simulink model "Two_Zone_MVDC_PSolver"  (R2025b)
settings: Solver=FixedStepDiscrete  StartTime=0.0  StopTime=30  FixedStep=TsELEC  RelTol=1e-3  EnableMultiTasking=on
InitFcn:
  | TsELEC = 25e-6;
  | Ts = 25e-6;
undefined symbols (not defined in the file or in its folder): DiscIntNeverNeededParam, ee_sli_rtmsupport, GABDA, GABDB, GBBDA, GBBDB, gcbh, GPPMA, GPPMB, GPPMC, SADA, SADB, SADC, SADD, SBDA, SBDB, SBDC, SCDA, SCDB, SCDC, SCDD, SDDA, SDDB, SDDC, SDDD, SDDE, TsCont
libraries: fl_lib x97, nesl_utility x73, ee_lib x48, simulink x3, slpidlib x3, eeSmAC1C x2, eePowerMeasurement x2, mcbeeMathTransformLib x2, eeTransforms x1
(part 3 of 4)

== system Two_Zone_MVDC_PSolver/PMM/Control ==
  Selector : Selector  InputPortWidth=2  IndexOptions=Index vector (dialog)  Indices=2  OutputSizes=1
  Selector1 : Selector  InputPortWidth=2  IndexOptions=Index vector (dialog)  Indices=1  OutputSizes=1
  Speed Control : Subsystem
  Torque Control : Subsystem
  Unit Delay1 : UnitDelay  SampleTime=Ts  HasFrameUpgradeWarning=on
  duty_cycle : Outport
  wires:
  Unit Delay1/1 -> duty_cycle/1
  [Nref1] -> Speed Control/1(Speed_Ref_PU)
  [pos_speed_1] -> Selector/1, Selector1/1
  Selector/1 -> Speed Control/2(Speed_Meas_PU)
  [Iab_meas1] -> Torque Control/2(Iab_Sim)
  Torque Control/1(Vabc_out_PU) -> Unit Delay1/1
  Selector1/1 -> Torque Control/3(Pos_Sim)
  Speed Control/1(IdqRef_PU) -> Torque Control/1(Idq_ref_PU)

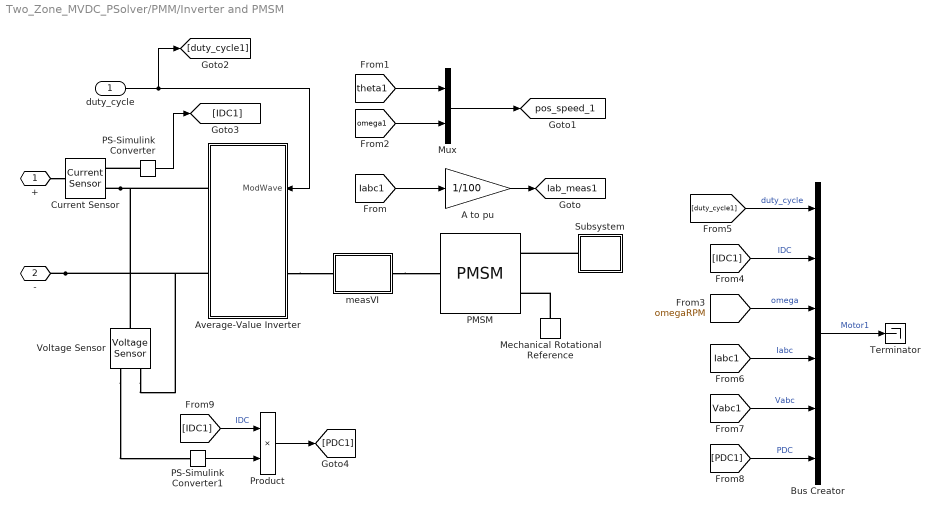
== system Two_Zone_MVDC_PSolver/PMM/Inverter and PMSM ==
  duty_cycle : Inport
  A to pu : Gain  Gain=1/100
  Average-Value Inverter : Subsystem
  Bus Creator : BusCreator  Inputs=6
  Current Sensor : fl_lib/Electrical/Electrical Sensors/Current Sensor
  Mechanical Rotational Reference : fl_lib/Mechanical/Rotational Elements/Mechanical Rotational Reference
  Mux : Mux  Inputs=2
  PMSM : ee_lib/Electromechanical/Permanent Magnet/PMSM  port_option=ee.enum.threePhasePort.composite  winding_type=ee.enum.statorconnection.wye  machine_param=ee.enum.pmsm.parameterization.constant  nPolePairs=1  pmflux_param=ee.enum.pmflux.fluxlinkage  pm_flux_linkage=3.15*4 Wb  torque_constant=0.18 N*m/A  back_emf_constant=0.18 V/(rad/s)  stator_param=ee.enum.statorparam.LdLqL0  Ld=0.0005 H  Lq=0.0009 H  idVec=[-200, 0, 200] A  iqVec=[-200, 0, 200] A  LdMatrix=0.0002 * ones(3, 3) H  LqMatrix=0.0002 * ones(3, 3) H  PmMatrix=0.1 * ones(3, 3) Wb  ktMatrix=0.18 * ones(3, 3) N*m/A  keMatrix=0.18 * ones(3, 3) V/(rad/s)  L0=0 H  Ls=0.0002 H  Lm=-0.00002 H  Ms=0.00002 H  Rs=0.001 Ohm  zero_sequence=ee.enum.park.zerosequence.exclude  axes_param=ee.enum.rotorangle.daxis  loss_param=ee.enum.ironloss.none  losses_oc=[0, 0, 0] W  losses_sc=[0, 0, 0] W  f_losses=60 Hz  Isc_losses=95 A  J=1 kg*m^2  lam=1 N*m/(rad/s)  i_d_specify=off  i_d_priority=None  i_d=0 A  i_d_nominal_specify=off  i_d_nominal_value=1  i_d_nominal_unit=A  i_q_specify=off  i_q_priority=None  i_q=0 A  i_q_nominal_specify=off  i_q_nominal_value=1  i_q_nominal_unit=A  torque_specify=off  torque_priority=None  torque=0 N*m  torque_nominal_specify=off  torque_nominal_value=1  torque_nominal_unit=N*m  angular_velocity_specify=off  angular_velocity_priority=High  angular_velocity=0 rpm  angular_velocity_nominal_specify=off  angular_velocity_nominal_value=1  angular_velocity_nominal_unit=rpm  angular_position_specify=off  angular_position_priority=High  angular_position=0 deg  angular_position_nominal_specify=off  angular_position_nominal_value=1  angular_position_nominal_unit=deg  alpha=3.93e-3 1/K  alpha_flux=-0.001 1/K  Tmeas=298.15 K  stator_thermal_mass=100 J/K  rotor_thermal_mass=200 J/K  Rm_percent_rotor=90  Rd_percent_rotor=30  temperatureA_specify=off  temperatureA_priority=High  temperatureA=25 degC  temperatureA_nominal_specify=off  temperatureA_nominal_value=1  temperatureA_nominal_unit=degC  temperatureB_specify=off  temperatureB_priority=High  temperatureB=25 degC  temperatureB_nominal_specify=off  temperatureB_nominal_value=1  temperatureB_nominal_unit=degC  temperatureC_specify=off  temperatureC_priority=High  temperatureC=25 degC  temperatureC_nominal_specify=off  temperatureC_nominal_value=1  temperatureC_nominal_unit=degC  temperatureR_specify=off  temperatureR_priority=High  temperatureR=25 degC  temperatureR_nominal_specify=off  temperatureR_nominal_value=1  temperatureR_nominal_unit=degC
      settings: InternalSimscapePortConfiguration="{\"Bottom\":[],\"Left\":[{\"id\":\"N\",\"label\":\"~\",\"type\":\"foundation.electrical.three_phase\"}],\"Right\":[{\"id\":\"R\",\"label\":\"R\",\"type\":\"foundation.mechanical.rotational.rotational\"},{\"id\":\"C\",\"label\":\"C\",\"type\":\"foundation.mechanical.rotational.rotational\"}],\"Top\":[]}"
  PS-Simulink Converter : nesl_utility/PS-Simulink Converter  PhysicalDomain=network_engine_domain  SubClassName=ps_output  LeftPortType=input  RightPortType=output  PseudoPeriodic=off  Frequencies=[]  VectorFormat=1-D array  Unit=inherit  AffineConversion=off
  PS-Simulink Converter1 : nesl_utility/PS-Simulink Converter  PhysicalDomain=network_engine_domain  SubClassName=ps_output  LeftPortType=input  RightPortType=output  PseudoPeriodic=off  Frequencies=[]  VectorFormat=1-D array  Unit=inherit  AffineConversion=off
  Product : Product
  Subsystem : Subsystem
  Terminator : Terminator
  Voltage Sensor : fl_lib/Electrical/Electrical Sensors/Voltage Sensor
  measVI : Subsystem
  + : PMIOPort  Side=Left
  - : PMIOPort  Port=2  Side=Left
  tag scope: Iab_meas1=global, pos_speed_1=global
  wires:
  duty_cycle/1 -> Average-Value Inverter/1(ModWave), [duty_cycle1]
  [IDC1] -> Product/1  "IDC"
  [PDC1] -> Bus Creator/6  "PDC"
  Product/1 -> [PDC1]
  PS-Simulink Converter1/1 -> Product/2
  A to pu/1 -> [Iab_meas1]
  [Iabc1] -> A to pu/1
  [theta1] -> Mux/1
  [omega1] -> Mux/2
  Mux/1 -> [pos_speed_1]
  PS-Simulink Converter/1 -> [IDC1]
  [duty_cycle1] -> Bus Creator/1  "duty_cycle"
  [IDC1] -> Bus Creator/2  "IDC"
  [omegaRPM] -> Bus Creator/3  "omega"
  Bus Creator/1 -> Terminator/1  "Motor1"
  [Iabc1] -> Bus Creator/4  "Iabc"
  [Vabc1] -> Bus Creator/5  "Vabc"
  connections:
  Voltage Sensor/RConn1 -- PS-Simulink Converter1/LConn1
  Mechanical Rotational Reference/LConn1 -- PMSM/RConn2
  Subsystem/RConn1 -- PMSM/RConn1
  Average-Value Inverter/LConn1 -- measVI/LConn1
  measVI/RConn1 -- PMSM/LConn1
  Current Sensor/RConn2 -- Voltage Sensor/LConn1 -- Average-Value Inverter/RConn1
  PS-Simulink Converter/LConn1 -- Current Sensor/RConn1
  +/RConn1 -- Current Sensor/LConn1
  -/RConn1 -- Voltage Sensor/RConn2 -- Average-Value Inverter/RConn2

== system Two_Zone_MVDC_PSolver/PMM/Speed Reference ==
  LPF : Subsystem
  Power Reference : simulink/Sources/Repeating Sequence Interpolated  OutValues=[0 0 0.5 0.5 -0.5 -0.5]  TimeValues=[0 5 10 15 25 100]  LookUpMeth=Interpolation-Use End Values  tsamp=TsELEC  OutMin=[]  OutMax=[]  OutDataTypeStr=double  OutputDataTypeScalingMode=double  OutDataType=fixdt(0,8)  OutScaling=2^-10
  tag scope: Nref1=global
  wires:
  Power Reference/1 -> LPF/1(u)
  LPF/1(y) -> [Nref1]

== system Two_Zone_MVDC_PSolver/PGM1/Gas turbine/ AC1C ==
  Constant1 : Constant  Value=0  SampleTime=TsCont
  Constant2 : Constant  Value=0  SampleTime=TsCont
  PS-Simulink Converter : nesl_utility/PS-Simulink Converter  PhysicalDomain=network_engine_domain  SubClassName=ps_output  LeftPortType=input  RightPortType=output  PseudoPeriodic=off  Frequencies=[]  VectorFormat=1-D array  Unit=inherit  AffineConversion=off
  PS-Simulink Converter1 : nesl_utility/PS-Simulink Converter  PhysicalDomain=network_engine_domain  SubClassName=ps_output  LeftPortType=input  RightPortType=output  PseudoPeriodic=off  Frequencies=[]  VectorFormat=1-D array  Unit=inherit  AffineConversion=off
  Rate Transition : RateTransition  OutPortSampleTime=TsELEC
  Rate Transition1 : RateTransition  OutPortSampleTime=TsCont
  Rate Transition2 : RateTransition  OutPortSampleTime=TsCont
  Repeating Sequence Interpolated2 : simulink/Sources/Repeating Sequence Interpolated  OutValues=[1 1 1]  TimeValues=[0 5 1000]  LookUpMeth=Interpolation-Use End Values  tsamp=TsCont  OutMin=[]  OutMax=[]  OutDataTypeStr=double  OutputDataTypeScalingMode=double  OutDataType=fixdt(0,8)  OutScaling=2^-10
  SM AC1C : eeSmAC1C/SM AC1C  E_FD0=1  Ts=TsCont  R_C=0  X_C=0  T_R=0  K_A=80  T_A=0.2  T_B=0  T_C=0  K_F=0.03  T_F=1.49  V_Amax=14.5  V_Amin=-14.5  E_FEmax=6.03  E_FEmin=-5.43  oelInputLocation=Unused  uelInputLocation=Unused  sclInputLocation=Unused  K_E=1  T_E=0.8  K_C=0.2  K_D=0.38  E_1=4.18  S_E_E1=0.1  E_2=3.14  S_E_E2=0.03  V_FEmax=99  V_Emin=0
      settings: LibrarySourceBlock=ee_sl_lib/SM Control/SM AC1C
  Simulink-PS Converter : nesl_utility/Simulink-PS Converter  PhysicalDomain=network_engine_domain  SubClassName=ps_input  LeftPortType=input  RightPortType=output  PseudoPeriodic=off  Frequencies=[]  NoiseDistribution=none  NoiseParameters=[]  Unit=1  AffineConversion=off  FilteringAndDerivatives=provide  SimscapeFilterOrder=1  InputFilterTimeConstant=0.001  UdotUserProvided=0
  Synchronous Machine Field Circuit (pu) : ee_lib/Electromechanical/Synchronous/Synchronous Machine Field Circuit  unit_option=ee.enum.unit.pu  SRated=36e6 V*A  FRated=60 Hz  fieldCircuitParameterization_option=ee.enum.sm.fieldparameterization.current  baseEfd=92.95 V  baseIfd=200 A  parameterization_option=ee.enum.sm.parameterization.standard  Ladu=1.66  Rfd=0.0006  Xl=0.15  Xd=1.81  Xdd=0.3  Xddd=0.23  d_option=ee.enum.circuit.open  Td0d=8 s  Tdd=1.3260 s  Td0dd=0.03 s  Tddd=0.0230 s
      settings: LogSimulationData=on  InternalSimscapePortConfiguration="{\"Bottom\":[],\"Left\":[{\"id\":\"Efd_pu\",\"label\":\"Efd_pu\",\"type\":\"input\"},{\"id\":\"Ifd_pu\",\"label\":\"Ifd_pu\",\"type\":\"output\"}],\"Right\":[{\"id\":\"fd_p\",\"label\":\"fd+\",\"type\":\"foundation.electrical.electrical\"},{\"id\":\"fd_n\",\"label\":\"fd-\",\"type\":\"foundation.electrical.electrical\"}],\"Top\":[]}"
  Terminal Voltage Measurement : ee_lib/Electromechanical/Synchronous/Synchronous Machine Measurement  output_idx=14
      settings: LogSimulationData=on  InternalSimscapePortConfiguration="{\"Bottom\":[],\"Left\":[{\"id\":\"pu_input\",\"label\":\"pu\",\"type\":\"input\"}],\"Right\":[{\"id\":\"pu_output\",\"label\":\"o\",\"type\":\"output\"}],\"Top\":[]}"
  Unit Delay : UnitDelay  InitialCondition=1.37673  SampleTime=-1  HasFrameUpgradeWarning=on
  pu : PMIOPort  Side=Left
  fd+ : PMIOPort  Port=2  Side=Right
  fd- : PMIOPort  Port=3  Side=Right
  wires:
  PS-Simulink Converter1/1 -> Unit Delay/1
  PS-Simulink Converter/1 -> Rate Transition1/1  "Vt1"
  Unit Delay/1 -> Rate Transition2/1  "Ifd1"
  Rate Transition/1 -> Simulink-PS Converter/1
  Repeating Sequence Interpolated2/1 -> SM AC1C/1
  Constant1/1 -> SM AC1C/2
  Rate Transition2/1 -> SM AC1C/10
  Rate Transition1/1 -> SM AC1C/3
  Constant2/1 -> SM AC1C/8, SM AC1C/7, SM AC1C/6, SM AC1C/5, SM AC1C/4, SM AC1C/9
  SM AC1C/1 -> Rate Transition/1
  connections:
  fd-/RConn1 -- Synchronous Machine Field Circuit (pu)/RConn2
  Synchronous Machine Field Circuit (pu)/RConn1 -- fd+/RConn1
  PS-Simulink Converter1/LConn1 -- Synchronous Machine Field Circuit (pu)/LConn2
  Simulink-PS Converter/RConn1 -- Synchronous Machine Field Circuit (pu)/LConn1
  pu/RConn1 -- Terminal Voltage Measurement/LConn1
  PS-Simulink Converter/LConn1 -- Terminal Voltage Measurement/RConn1

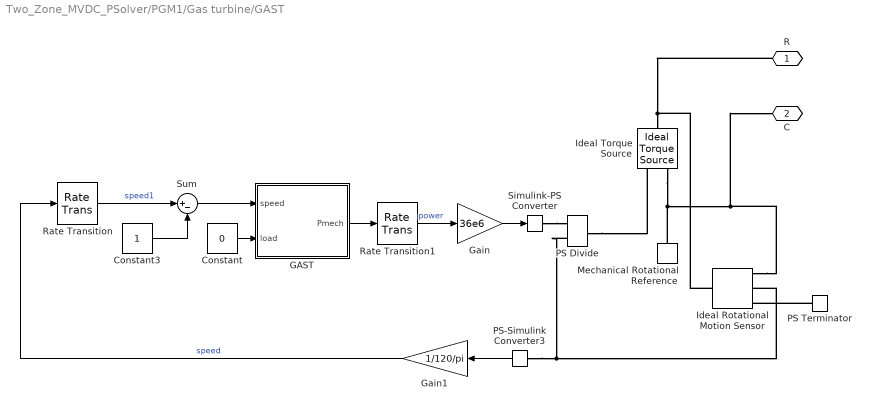
== system Two_Zone_MVDC_PSolver/PGM1/Gas turbine/GAST ==
  Constant : Constant  Value=0  SampleTime=TsCont
  Constant3 : Constant  SampleTime=TsCont
  GAST : Subsystem  mask{R=0.01, T1=0.005, T2=0.04, T3=0.1, AT=0.9, Kt=2, Vmax=1, Vmin=0, Dturb=0.03}
  Gain : Gain  Gain=36e6
  Gain1 : Gain  Gain=1/120/pi
  Ideal Rotational Motion Sensor : fl_lib/Mechanical/Mechanical Sensors/Ideal Rotational Motion Sensor  reference=foundation.enum.MeasurementReference.difference  acceleration_port=false  velocity_port=true  position_port=true  wrap_angle=simscape.enum.onoff.off  offset=0 rad
  Ideal Torque Source : fl_lib/Mechanical/Mechanical Sources/Ideal Torque Source
  Mechanical Rotational Reference : fl_lib/Mechanical/Rotational Elements/Mechanical Rotational Reference
  PS Divide : fl_lib/Physical Signals/Functions/PS Divide
  PS Terminator : fl_lib/Physical Signals/Sinks/PS Terminator
  PS-Simulink Converter3 : nesl_utility/PS-Simulink Converter  PhysicalDomain=network_engine_domain  SubClassName=ps_output  LeftPortType=input  RightPortType=output  PseudoPeriodic=off  Frequencies=[]  VectorFormat=1-D array  Unit=inherit  AffineConversion=off
  Rate Transition : RateTransition  Deterministic=off  OutPortSampleTime=TsCont
  Rate Transition1 : RateTransition  Deterministic=off  InitialCondition=2000/3/60*2*pi  OutPortSampleTime=Ts
  Simulink-PS Converter : nesl_utility/Simulink-PS Converter  PhysicalDomain=network_engine_domain  SubClassName=ps_input  LeftPortType=input  RightPortType=output  PseudoPeriodic=off  Frequencies=[]  NoiseDistribution=none  NoiseParameters=[]  Unit=W  AffineConversion=off  FilteringAndDerivatives=provide  SimscapeFilterOrder=1  InputFilterTimeConstant=0.001  UdotUserProvided=0
  Sum : Sum  Inputs=|+-
  R : PMIOPort  Side=Right
  C : PMIOPort  Port=2  Side=Right
  wires:
  Constant3/1 -> Sum/2
  Gain1/1 -> Rate Transition/1  "speed"
  GAST/1(Pmech) -> Rate Transition1/1
  Constant/1 -> GAST/2(load)
  Rate Transition1/1 -> Gain/1  "power"
  Rate Transition/1 -> Sum/1  "speed1"
  Sum/1 -> GAST/1(speed)
  Gain/1 -> Simulink-PS Converter/1
  PS-Simulink Converter3/1 -> Gain1/1
  connections:
  Ideal Rotational Motion Sensor/RConn2 -- PS-Simulink Converter3/LConn1 -- PS Divide/LConn2
  PS Terminator/LConn1 -- Ideal Rotational Motion Sensor/RConn3
  Ideal Torque Source/RConn2 -- Mechanical Rotational Reference/LConn1 -- C/RConn1 -- Ideal Rotational Motion Sensor/RConn1
  PS Divide/RConn1 -- Ideal Torque Source/RConn1
  Simulink-PS Converter/RConn1 -- PS Divide/LConn1
  R/RConn1 -- Ideal Rotational Motion Sensor/LConn1 -- Ideal Torque Source/LConn1

== system Two_Zone_MVDC_PSolver/PGM2/Gas turbine/ AC1C ==
  Constant1 : Constant  Value=0  SampleTime=TsCont
  Constant2 : Constant  Value=0  SampleTime=TsCont
  PS-Simulink Converter : nesl_utility/PS-Simulink Converter  PhysicalDomain=network_engine_domain  SubClassName=ps_output  LeftPortType=input  RightPortType=output  PseudoPeriodic=off  Frequencies=[]  VectorFormat=1-D array  Unit=inherit  AffineConversion=off
  PS-Simulink Converter1 : nesl_utility/PS-Simulink Converter  PhysicalDomain=network_engine_domain  SubClassName=ps_output  LeftPortType=input  RightPortType=output  PseudoPeriodic=off  Frequencies=[]  VectorFormat=1-D array  Unit=inherit  AffineConversion=off
  Rate Transition : RateTransition  OutPortSampleTime=TsELEC
  Rate Transition1 : RateTransition  OutPortSampleTime=TsCont
  Rate Transition2 : RateTransition  OutPortSampleTime=TsCont
  Repeating Sequence Interpolated2 : simulink/Sources/Repeating Sequence Interpolated  OutValues=[1 1 1]  TimeValues=[0 5 1000]  LookUpMeth=Interpolation-Use End Values  tsamp=TsCont  OutMin=[]  OutMax=[]  OutDataTypeStr=double  OutputDataTypeScalingMode=double  OutDataType=fixdt(0,8)  OutScaling=2^-10
  SM AC1C : eeSmAC1C/SM AC1C  E_FD0=1  Ts=TsCont  R_C=0  X_C=0  T_R=0  K_A=80  T_A=0.2  T_B=0  T_C=0  K_F=0.03  T_F=1.49  V_Amax=14.5  V_Amin=-14.5  E_FEmax=6.03  E_FEmin=-5.43  oelInputLocation=Unused  uelInputLocation=Unused  sclInputLocation=Unused  K_E=1  T_E=0.8  K_C=0.2  K_D=0.38  E_1=4.18  S_E_E1=0.1  E_2=3.14  S_E_E2=0.03  V_FEmax=99  V_Emin=0
      settings: LibrarySourceBlock=ee_sl_lib/SM Control/SM AC1C
  Simulink-PS Converter : nesl_utility/Simulink-PS Converter  PhysicalDomain=network_engine_domain  SubClassName=ps_input  LeftPortType=input  RightPortType=output  PseudoPeriodic=off  Frequencies=[]  NoiseDistribution=none  NoiseParameters=[]  Unit=1  AffineConversion=off  FilteringAndDerivatives=provide  SimscapeFilterOrder=1  InputFilterTimeConstant=0.001  UdotUserProvided=0
  Synchronous Machine Field Circuit (pu) : ee_lib/Electromechanical/Synchronous/Synchronous Machine Field Circuit  unit_option=ee.enum.unit.pu  SRated=36e6 V*A  FRated=60 Hz  fieldCircuitParameterization_option=ee.enum.sm.fieldparameterization.current  baseEfd=92.95 V  baseIfd=200 A  parameterization_option=ee.enum.sm.parameterization.standard  Ladu=1.66  Rfd=0.0006  Xl=0.15  Xd=1.81  Xdd=0.3  Xddd=0.23  d_option=ee.enum.circuit.open  Td0d=8 s  Tdd=1.3260 s  Td0dd=0.03 s  Tddd=0.0230 s
      settings: LogSimulationData=on  InternalSimscapePortConfiguration="{\"Bottom\":[],\"Left\":[{\"id\":\"Efd_pu\",\"label\":\"Efd_pu\",\"type\":\"input\"},{\"id\":\"Ifd_pu\",\"label\":\"Ifd_pu\",\"type\":\"output\"}],\"Right\":[{\"id\":\"fd_p\",\"label\":\"fd+\",\"type\":\"foundation.electrical.electrical\"},{\"id\":\"fd_n\",\"label\":\"fd-\",\"type\":\"foundation.electrical.electrical\"}],\"Top\":[]}"
  Terminal Voltage Measurement : ee_lib/Electromechanical/Synchronous/Synchronous Machine Measurement  output_idx=14
      settings: LogSimulationData=on  InternalSimscapePortConfiguration="{\"Bottom\":[],\"Left\":[{\"id\":\"pu_input\",\"label\":\"pu\",\"type\":\"input\"}],\"Right\":[{\"id\":\"pu_output\",\"label\":\"o\",\"type\":\"output\"}],\"Top\":[]}"
  Unit Delay : UnitDelay  InitialCondition=1.37673  SampleTime=-1  HasFrameUpgradeWarning=on
  pu : PMIOPort  Side=Left
  fd+ : PMIOPort  Port=2  Side=Right
  fd- : PMIOPort  Port=3  Side=Right
  wires:
  SM AC1C/1 -> Rate Transition/1
  PS-Simulink Converter1/1 -> Unit Delay/1
  Repeating Sequence Interpolated2/1 -> SM AC1C/1
  PS-Simulink Converter/1 -> Rate Transition1/1  "Vt1"
  Unit Delay/1 -> Rate Transition2/1  "Ifd1"
  Constant1/1 -> SM AC1C/2
  Rate Transition/1 -> Simulink-PS Converter/1
  Rate Transition1/1 -> SM AC1C/3
  Rate Transition2/1 -> SM AC1C/10
  Constant2/1 -> SM AC1C/8, SM AC1C/7, SM AC1C/6, SM AC1C/5, SM AC1C/4, SM AC1C/9
  connections:
  fd-/RConn1 -- Synchronous Machine Field Circuit (pu)/RConn2
  Synchronous Machine Field Circuit (pu)/RConn1 -- fd+/RConn1
  PS-Simulink Converter1/LConn1 -- Synchronous Machine Field Circuit (pu)/LConn2
  Simulink-PS Converter/RConn1 -- Synchronous Machine Field Circuit (pu)/LConn1
  pu/RConn1 -- Terminal Voltage Measurement/LConn1
  PS-Simulink Converter/LConn1 -- Terminal Voltage Measurement/RConn1

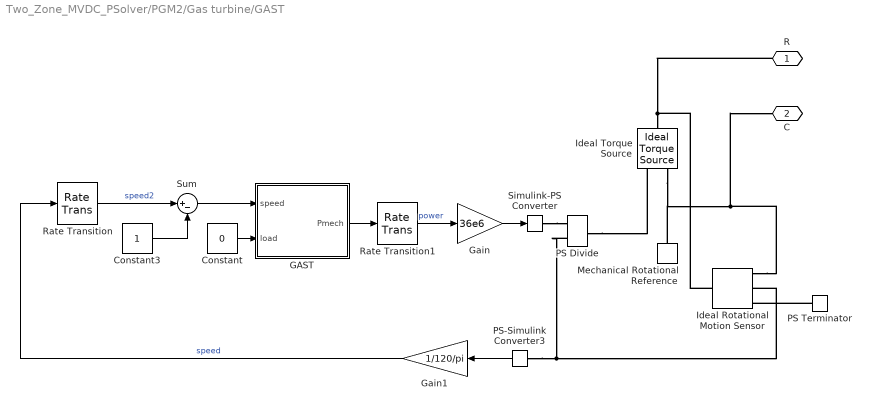
== system Two_Zone_MVDC_PSolver/PGM2/Gas turbine/GAST ==
  Constant : Constant  Value=0  SampleTime=TsCont
  Constant3 : Constant  SampleTime=TsCont
  GAST : Subsystem  mask{R=0.01, T1=0.005, T2=0.04, T3=0.1, AT=0.9, Kt=2, Vmax=1, Vmin=0, Dturb=0.03}
  Gain : Gain  Gain=36e6
  Gain1 : Gain  Gain=1/120/pi
  Ideal Rotational Motion Sensor : fl_lib/Mechanical/Mechanical Sensors/Ideal Rotational Motion Sensor  reference=foundation.enum.MeasurementReference.difference  acceleration_port=false  velocity_port=true  position_port=true  wrap_angle=simscape.enum.onoff.off  offset=0 rad
  Ideal Torque Source : fl_lib/Mechanical/Mechanical Sources/Ideal Torque Source
  Mechanical Rotational Reference : fl_lib/Mechanical/Rotational Elements/Mechanical Rotational Reference
  PS Divide : fl_lib/Physical Signals/Functions/PS Divide
  PS Terminator : fl_lib/Physical Signals/Sinks/PS Terminator
  PS-Simulink Converter3 : nesl_utility/PS-Simulink Converter  PhysicalDomain=network_engine_domain  SubClassName=ps_output  LeftPortType=input  RightPortType=output  PseudoPeriodic=off  Frequencies=[]  VectorFormat=1-D array  Unit=inherit  AffineConversion=off
  Rate Transition : RateTransition  Deterministic=off  OutPortSampleTime=TsCont
  Rate Transition1 : RateTransition  Deterministic=off  InitialCondition=2000/3/60*2*pi  OutPortSampleTime=Ts
  Simulink-PS Converter : nesl_utility/Simulink-PS Converter  PhysicalDomain=network_engine_domain  SubClassName=ps_input  LeftPortType=input  RightPortType=output  PseudoPeriodic=off  Frequencies=[]  NoiseDistribution=none  NoiseParameters=[]  Unit=W  AffineConversion=off  FilteringAndDerivatives=provide  SimscapeFilterOrder=1  InputFilterTimeConstant=0.001  UdotUserProvided=0
  Sum : Sum  Inputs=|+-
  R : PMIOPort  Side=Right
  C : PMIOPort  Port=2  Side=Right
  wires:
  Constant3/1 -> Sum/2
  Gain1/1 -> Rate Transition/1  "speed"
  GAST/1(Pmech) -> Rate Transition1/1
  Constant/1 -> GAST/2(load)
  Rate Transition1/1 -> Gain/1  "power"
  Rate Transition/1 -> Sum/1  "speed2"
  Sum/1 -> GAST/1(speed)
  Gain/1 -> Simulink-PS Converter/1
  PS-Simulink Converter3/1 -> Gain1/1
  connections:
  PS Divide/LConn2 -- Ideal Rotational Motion Sensor/RConn2 -- PS-Simulink Converter3/LConn1
  PS Terminator/LConn1 -- Ideal Rotational Motion Sensor/RConn3
  Ideal Rotational Motion Sensor/RConn1 -- Mechanical Rotational Reference/LConn1 -- Ideal Torque Source/RConn2 -- C/RConn1
  PS Divide/RConn1 -- Ideal Torque Source/RConn1
  Simulink-PS Converter/RConn1 -- PS Divide/LConn1
  R/RConn1 -- Ideal Torque Source/LConn1 -- Ideal Rotational Motion Sensor/LConn1

== system Two_Zone_MVDC_PSolver/PMM/Control/Speed Control ==
  Speed_Ref_PU : Inport
  Speed_Meas_PU : Inport  Port=2
  Id_ref : Constant  Value=0  OutDataTypeStr=Inherit: Inherit via back propagation  SampleTime=Ts
  Mux1 : Mux  Inputs=2
  PI_Controller_Speed : Subsystem
  IdqRef_PU : Outport  VectorParamsAs1DForOutWhenUnconnected=off
  wires:
  PI_Controller_Speed/1(Iq_ref) -> Mux1/2
  Id_ref/1 -> Mux1/1
  Speed_Ref_PU/1 -> PI_Controller_Speed/1(N_ref)
  Speed_Meas_PU/1 -> PI_Controller_Speed/2(N_fb)
  Mux1/1 -> IdqRef_PU/1

== system Two_Zone_MVDC_PSolver/PMM/Control/Torque Control ==
  Idq_ref_PU : Inport
  Iab_Sim : Inport  Port=2
  Pos_Sim : Inport  Port=3
  Control_System : Subsystem
  Gain : Gain
  Selector : Selector  InputPortWidth=3  IndexOptions=Index vector (dialog)  Indices=[1 2]  OutputSizes=1
  Vabc_out_PU : Outport  VectorParamsAs1DForOutWhenUnconnected=off
  wires:
  Selector/1 -> Control_System/1(Iab_meas_PU)
  Control_System/1(Vabc in PU) -> Vabc_out_PU/1
  Pos_Sim/1 -> Gain/1
  Iab_Sim/1 -> Selector/1
  Idq_ref_PU/1 -> Control_System/3(Idq_ref_PU)
  Gain/1 -> Control_System/2(Pos_PU)

== system Two_Zone_MVDC_PSolver/PMM/Inverter and PMSM/Average-Value Inverter ==
  ModWave : Inport
  Average-Value Voltage Source Converter (Three-Phase) : ee_lib/Semiconductors & Converters/Converters/Average-Value Voltage Source Converter (Three-Phase)  port_option=ee.enum.threePhasePort.composite  frequency_option=ee.enum.converters.frequency.variable  input_option=ee.enum.converters.inputOption.ModWave  FRated=60 Hz  losses_parameterization=ee.enum.converters.losses.fixed  Pfixed=1 W  ks=0.01  kc1=1.7 V  kc2=0.01 Ohm  Ploss_vect=[100, 800, 1870, 3250, 4900] W  Irms_vect=[10, 100, 200, 300, 400] A  Vdc_nom=300 V  thermal_mass=30000 J/K  temperature_specify=off  temperature_priority=High  temperature=298.15 K  temperature_nominal_specify=off  temperature_nominal_value=1  temperature_nominal_unit=K
      settings: InternalSimscapePortConfiguration="{\"Bottom\":[],\"Left\":[{\"id\":\"ModWave\",\"label\":\"ModWave\",\"type\":\"input\"},{\"id\":\"N\",\"label\":\"~\",\"type\":\"foundation.electrical.three_phase\"}],\"Right\":[{\"id\":\"p\",\"label\":\"+\",\"type\":\"foundation.electrical.electrical\"},{\"id\":\"n\",\"label\":\"-\",\"type\":\"foundation.electrical.electrical\"}],\"Top\":[]}"
  Simulink-PS Converter : nesl_utility/Simulink-PS Converter  PhysicalDomain=network_engine_domain  SubClassName=ps_input  LeftPortType=input  RightPortType=output  PseudoPeriodic=off  Frequencies=[]  NoiseDistribution=none  NoiseParameters=[]  Unit=1  AffineConversion=off  FilteringAndDerivatives=zero  SimscapeFilterOrder=1  InputFilterTimeConstant=0.001  UdotUserProvided=0
  + : PMIOPort  Side=Right
  ~ : PMIOPort  Port=2  Side=Left
  - : PMIOPort  Port=3  Side=Right
  wires:
  ModWave/1 -> Simulink-PS Converter/1
  connections:
  Simulink-PS Converter/RConn1 -- Average-Value Voltage Source Converter (Three-Phase)/LConn1
  Average-Value Voltage Source Converter (Three-Phase)/RConn2 -- -/RConn1
  Average-Value Voltage Source Converter (Three-Phase)/RConn1 -- +/RConn1
  Average-Value Voltage Source Converter (Three-Phase)/LConn2 -- ~/RConn1

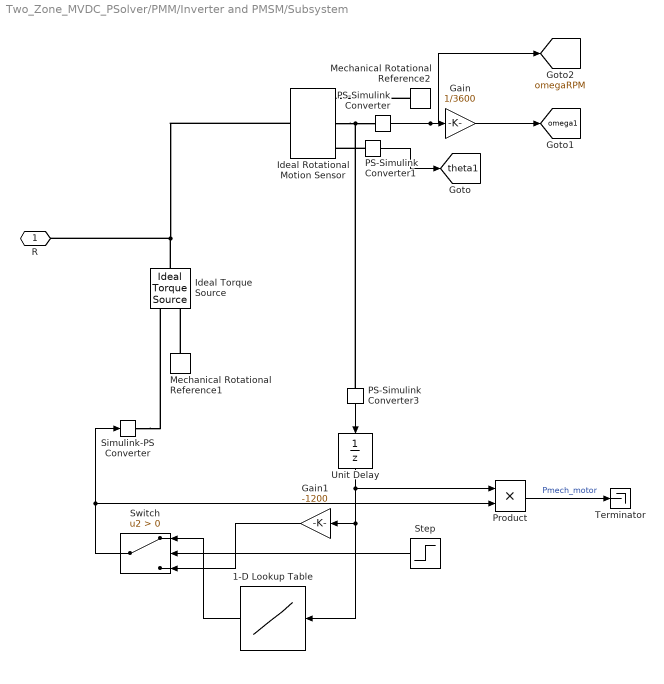
== system Two_Zone_MVDC_PSolver/PMM/Inverter and PMSM/Subsystem ==
  1-D Lookup Table : Lookup_n-D  NumberOfTableDimensions=1  BreakpointsForDimension1=[-120*pi 0 50*pi 120*pi]/2  Table=[120*pi*1200 50*pi*1200 0 -120*pi*1200]/2  InternalRulePriority=Speed  RndMeth=Simplest
  Gain : Gain  Gain=1/3600
  Gain1 : Gain  Gain=-1200
  Ideal Rotational Motion Sensor : fl_lib/Mechanical/Mechanical Sensors/Ideal Rotational Motion Sensor  reference=foundation.enum.MeasurementReference.difference  acceleration_port=false  velocity_port=true  position_port=true  wrap_angle=simscape.enum.onoff.off  offset=0 rad
  Ideal Torque Source : fl_lib/Mechanical/Mechanical Sources/Ideal Torque Source
  Mechanical Rotational Reference1 : fl_lib/Mechanical/Rotational Elements/Mechanical Rotational Reference
  Mechanical Rotational Reference2 : fl_lib/Mechanical/Rotational Elements/Mechanical Rotational Reference
  PS-Simulink Converter : nesl_utility/PS-Simulink Converter  PhysicalDomain=network_engine_domain  SubClassName=ps_output  LeftPortType=input  RightPortType=output  PseudoPeriodic=off  Frequencies=[]  VectorFormat=1-D array  Unit=rpm  AffineConversion=off
  PS-Simulink Converter1 : nesl_utility/PS-Simulink Converter  PhysicalDomain=network_engine_domain  SubClassName=ps_output  LeftPortType=input  RightPortType=output  PseudoPeriodic=off  Frequencies=[]  VectorFormat=1-D array  Unit=inherit  AffineConversion=off
  PS-Simulink Converter3 : nesl_utility/PS-Simulink Converter  PhysicalDomain=network_engine_domain  SubClassName=ps_output  LeftPortType=input  RightPortType=output  PseudoPeriodic=off  Frequencies=[]  VectorFormat=1-D array  Unit=inherit  AffineConversion=off
  Product : Product
  Simulink-PS Converter : nesl_utility/Simulink-PS Converter  PhysicalDomain=network_engine_domain  SubClassName=ps_input  LeftPortType=input  RightPortType=output  PseudoPeriodic=off  Frequencies=[]  NoiseDistribution=none  NoiseParameters=[]  Unit=1  AffineConversion=off  FilteringAndDerivatives=provide  SimscapeFilterOrder=1  InputFilterTimeConstant=0.001  UdotUserProvided=0
  Step : Step  Time=12.5  SampleTime=TsELEC
  Switch : Switch  Criteria=u2 > Threshold  SaturateOnIntegerOverflow=off  InputSameDT=off
  Terminator : Terminator
  Unit Delay : UnitDelay  SampleTime=-1  HasFrameUpgradeWarning=on
  "R " : PMIOPort  Side=Right
  tag scope: omega1=global, omegaRPM=global, theta1=global
  wires:
  Product/1 -> Terminator/1  "Pmech_motor"
  PS-Simulink Converter/1 -> Gain/1, [omegaRPM]
  Gain/1 -> [omega1]
  PS-Simulink Converter1/1 -> [theta1]
  1-D Lookup Table/1 -> Switch/1
  Switch/1 -> Simulink-PS Converter/1, Product/2
  Step/1 -> Switch/2
  Unit Delay/1 -> 1-D Lookup Table/1, Gain1/1, Product/1
  Gain1/1 -> Switch/3
  PS-Simulink Converter3/1 -> Unit Delay/1
  connections:
  Ideal Rotational Motion Sensor/LConn1 -- Ideal Torque Source/LConn1 -- "R "/RConn1
  Ideal Rotational Motion Sensor/RConn2 -- PS-Simulink Converter3/LConn1 -- PS-Simulink Converter/LConn1
  PS-Simulink Converter1/LConn1 -- Ideal Rotational Motion Sensor/RConn3
  Mechanical Rotational Reference2/LConn1 -- Ideal Rotational Motion Sensor/RConn1
  Mechanical Rotational Reference1/LConn1 -- Ideal Torque Source/RConn2
  Simulink-PS Converter/RConn1 -- Ideal Torque Source/RConn1

== system Two_Zone_MVDC_PSolver/PMM/Inverter and PMSM/measVI ==
  Current Sensor (Three-Phase) : ee_lib/Sensors & Transducers/Current Sensor (Three-Phase)
  Line Voltage Sensor (Three-Phase) : ee_lib/Sensors & Transducers/Line Voltage Sensor (Three-Phase)
  PS-Simulink Converter2 : nesl_utility/PS-Simulink Converter  PhysicalDomain=network_engine_domain  SubClassName=ps_output  LeftPortType=input  RightPortType=output  PseudoPeriodic=off  Frequencies=[]  VectorFormat=1-D array  Unit=inherit  AffineConversion=off
  PS-Simulink Converter3 : nesl_utility/PS-Simulink Converter  PhysicalDomain=network_engine_domain  SubClassName=ps_output  LeftPortType=input  RightPortType=output  PseudoPeriodic=off  Frequencies=[]  VectorFormat=1-D array  Unit=inherit  AffineConversion=off
  ~1 : PMIOPort  Side=Left
  ~2 : PMIOPort  Port=2  Side=Right
  tag scope: Iabc1=global, Vabc1=global
  wires:
  PS-Simulink Converter2/1 -> [Vabc1]  "Vabc 1"
  PS-Simulink Converter3/1 -> [Iabc1]  "Iabc 1"
  connections:
  Current Sensor (Three-Phase)/RConn1 -- PS-Simulink Converter3/LConn1
  PS-Simulink Converter2/LConn1 -- Line Voltage Sensor (Three-Phase)/RConn1
  Current Sensor (Three-Phase)/RConn2 -- ~2/RConn1
  Line Voltage Sensor (Three-Phase)/LConn1 -- ~1/RConn1 -- Current Sensor (Three-Phase)/LConn1

== system Two_Zone_MVDC_PSolver/PMM/Speed Reference/LPF ==
  u : Inport
  Discrete-Time Integrator : DiscreteIntegrator  gainval=20  SampleTime=Ts  ICPrevOutput=DiscIntNeverNeededParam  ICPrevScaledInput=DiscIntNeverNeededParam
  Sum : Sum  Inputs=|+-
  y : Outport
  wires:
  Sum/1 -> Discrete-Time Integrator/1
  Discrete-Time Integrator/1 -> y/1, Sum/2
  u/1 -> Sum/1

== system Two_Zone_MVDC_PSolver/PGM1/Gas turbine/GAST/GAST ==
  speed : Inport
  load : Inport  Port=2
  Constant : Constant  Value=AT  SampleTime=TsCont
  Gain : Gain  Gain=Dturb
  Gain1 : Gain  Gain=1/R
  Gain2 : Gain  Gain=Kt
  Min : MinMax  Inputs=2
  Subsystem : Subsystem  mask{T=T1, VMAX=Vmax, VMIN=Vmin}
  Subsystem1 : Subsystem  mask{T=T2, VMAX=Inf, VMIN=-Inf}
  Subsystem2 : Subsystem  mask{T=T3, VMAX=Inf, VMIN=-Inf}
  Sum : Sum  Inputs=-+|
  Sum1 : Sum  Inputs=-+|
  Sum2 : Sum  Inputs=|-+
  Sum3 : Sum  Inputs=|++
  Pmech : Outport
  wires:
  Gain1/1 -> Sum/1
  Min/1 -> Subsystem/1(u)
  Gain/1 -> Sum1/1
  Constant/1 -> Sum2/2, Sum3/2
  Sum2/1 -> Gain2/1
  Sum/1 -> Min/1
  Subsystem1/1(y) -> Subsystem2/1(u), Sum1/2
  Subsystem/1(y) -> Subsystem1/1(u)
  speed/1 -> Gain1/1, Gain/1
  Gain2/1 -> Sum3/1
  Sum3/1 -> Min/2
  Subsystem2/1(y) -> Sum2/1
  load/1 -> Sum/2
  Sum1/1 -> Pmech/1  "Pmech2"

== system Two_Zone_MVDC_PSolver/PGM2/Gas turbine/GAST/GAST ==
  speed : Inport
  load : Inport  Port=2
  Constant : Constant  Value=AT  SampleTime=TsCont
  Gain : Gain  Gain=Dturb
  Gain1 : Gain  Gain=1/R
  Gain2 : Gain  Gain=Kt
  Min : MinMax  Inputs=2
  Subsystem : Subsystem  mask{T=T1, VMAX=Vmax, VMIN=Vmin}
  Subsystem1 : Subsystem  mask{T=T2, VMAX=Inf, VMIN=-Inf}
  Subsystem2 : Subsystem  mask{T=T3, VMAX=Inf, VMIN=-Inf}
  Sum : Sum  Inputs=-+|
  Sum1 : Sum  Inputs=-+|
  Sum2 : Sum  Inputs=|-+
  Sum3 : Sum  Inputs=|++
  Pmech : Outport
  wires:
  Gain1/1 -> Sum/1
  Min/1 -> Subsystem/1(u)
  Gain/1 -> Sum1/1
  Constant/1 -> Sum2/2, Sum3/2
  Sum2/1 -> Gain2/1
  Sum/1 -> Min/1
  Subsystem1/1(y) -> Subsystem2/1(u), Sum1/2
  Subsystem/1(y) -> Subsystem1/1(u)
  speed/1 -> Gain1/1, Gain/1
  Gain2/1 -> Sum3/1
  Sum3/1 -> Min/2
  Subsystem2/1(y) -> Sum2/1
  load/1 -> Sum/2
  Sum1/1 -> Pmech/1  "Pmech1"

== system Two_Zone_MVDC_PSolver/PMM/Control/Speed Control/PI_Controller_Speed ==
  N_ref : Inport
  N_fb : Inport  Port=2
  Constant : Constant  Value=0  SampleTime=Ts
  Discrete PID Controller : slpidlib/PID Controller  Controller=PID  Form=Parallel  TimeDomain=Discrete-time  UseExternalTs=off  SampleTime=Ts  IntegratorMethod=Forward Euler  FilterMethod=Forward Euler  ControllerParametersSource=internal  P=500  I=200*10  UseKiTs=off  D=0  UseExternalDerivativeSource=off  N=100  UseFilter=on  TunerSelectOption=Transfer Function Based (PID Tuner App)  InitialConditionSource=internal  InitialConditionForIntegrator=0  InitialConditionForFilter=0  DifferentiatorICPrevScaledInput=0  ExternalReset=either  TrackingMode=off  Kt=1  LimitOutput=off  SatLimitsSource=internal  UpperSaturationLimit=inf  LowerSaturationLimit=-inf  LinearizeAsGain=off  AntiWindupMode=none  Kb=1  LimitIntegrator=off  UpperIntegratorSaturationLimit=inf  LowerIntegratorSaturationLimit=-inf  POutMin=[]  POutMax=[]  IOutMin=[]  IOutMax=[]  DOutMin=[]  DOutMax=[]  NOutMin=[]  NOutMax=[]  SumOutMin=[]  SumOutMax=[]  SaturationOutMin=[]  SaturationOutMax=[]  PParamMin=[]  PParamMax=[]  IParamMin=[]  IParamMax=[]  DParamMin=[]  DParamMax=[]  NParamMin=[]  NParamMax=[]  KbParamMin=[]  KbParamMax=[]  KtParamMin=[]  KtParamMax=[]  KbOutMin=[]  KbOutMax=[]  KtOutMin=[]  KtOutMax=[]  IntegratorOutMin=[]  IntegratorOutMax=[]  FilterOutMin=[]  FilterOutMax=[]  SumI1OutMin=[]  SumI1OutMax=[]  SumI2OutMin=[]  SumI2OutMax=[]  SumI3OutMin=[]  SumI3OutMax=[]  SumI4OutMin=[]  SumI4OutMax=[]  SumDOutMin=[]  SumDOutMax=[]  DifferentiatorOutMin=[]  DifferentiatorOutMax=[]  FilterDiffOutCoefMin=[]  FilterDiffOutCoefMax=[]  ReciprocalOutMin=[]  ReciprocalOutMax=[]  SumDenOutMin=[]  SumDenOutMax=[]  SumNumOutMin=[]  SumNumOutMax=[]  DivideOutMin=[]  DivideOutMax=[]  UdiffTsProdOutMin=[]  UdiffTsProdOutMax=[]  NTsProdOutMin=[]  NTsProdOutMax=[]  UintegralTsProdOutMin=[]  UintegralTsProdOutMax=[]  UngainTsProdOutMin=[]  UngainTsProdOutMax=[]  ClampingZeroOutDataTypeStr=Inherit: Inherit via back propagation  ClampingZeroOutMin=[]  ClampingZeroOutMax=[]  FilterDenConstantOutDataTypeStr=Inherit: Inherit via back propagation  FilterDenConstantOutMin=[]  FilterDenConstantOutMax=[]  PCopyOutDataTypeStr=Inherit: Inherit via back propagation  PCopyOutMin=[]  PCopyOutMax=[]  NCopyOutDataTypeStr=Inherit: Inherit via back propagation  NCopyOutMin=[]  NCopyOutMax=[]  IntegratorContinuousStateAttributes=''  IntegratorStateMustResolveToSignalObject=off  IntegratorRTWStateStorageClass=Auto  FilterContinuousStateAttributes=''  FilterStateMustResolveToSignalObject=off  FilterRTWStateStorageClass=Auto  ParallelPVariant=InternalParameters  IdealPVariant=Disabled  IVariant=InternalParameters  DVariant=InternalParameters  IntegratorVariant=Discrete  SatVariant=Disabled  AWVariant=Passthrough  PCopyVariant=Disabled  TRVariant=Disabled  FdbkBlocksVariant=Forward  IdealPFdbkVariant=Disabled  SatFdbkVariant=Disabled  DerivativeFilterVariant=ForwardEulerFilter  NVariant=InternalParameters  NCopyVariant=Disabled  FilterICVariant=InternalICsFilter  IntegratorICVariant=InternalICs  ExternalResetVariant=ExternalReset  TRSumVariant=Passthrough  SumFdbkVariant=Disabled  SumVariant=Sum_PID  TsampFilterVariant=InternalTs  TsampNgainVariant=Passthrough  TsampIntegralVariant=Disabled_SignalSpec  ExternalSaturationOutDataTypeStr=Inherit: Same as second input  DerivativeSourceVariant=ErrorSignal  PreIntVariant=InternalPreInt
  Sum : Sum  Inputs=|+-  RndMeth=Round
  Iq_ref : Outport  VectorParamsAs1DForOutWhenUnconnected=off
  wires:
  Constant/1 -> Discrete PID Controller/2
  Discrete PID Controller/1 -> Iq_ref/1
  Sum/1 -> Discrete PID Controller/1
  N_ref/1 -> Sum/1
  N_fb/1 -> Sum/2

== system Two_Zone_MVDC_PSolver/PMM/Control/Torque Control/Control_System ==
  Iab_meas_PU : Inport
  Pos_PU : Inport  Port=2
  Idq_ref_PU : Inport  Port=3
  Clarke Transform : mcbeeMathTransformLib/Clarke Transform  PowerInvariant=off  UseWithEmbedded=off  PhaseInput=Two inputs
  Clarke to Park Angle Transform : mcbeeMathTransformLib/Clarke to Park Angle Transform  AxisAlignment=D-axis  UseWithEmbedded=off  PhaseInput=Two inputs  ThetaInput=Sine and Cosine electrical position  AngleInput=Per-unit  N_points=1024
  Constant : Constant  Value=0  SampleTime=Ts
  Constant1 : Constant  Value=sqrt(3)  SampleTime=Ts
  Current_Controllers : Subsystem
  Demux1 : Demux  Outputs=3
  Inverse Park Transform : eeTransforms/Inverse Park Transform  AxisAlignment=D-axis  PowerInvariant=off
  Mux : Mux  Inputs=3
  "PWM Generator (Three-phase, Two-level)" : Subsystem  LoadFcn=ee_sli_rtmsupport( 'loadfcn', gcbh );  mask(PWM Generator (three-phase, two-level)){PWMMode=Continuous PWM (CPWM), CPWMMode=SVM: space vector modulation, DPWMMode=60 DPWM: 60 degree discontinuous PWM, SamplingMode=Natural, fsw=1/Ts/10, Ts=Ts}
      mask prompts: PWMMode "physmod:ee:library:comments:control:eePwmGeneratorTwoLevel:PWMMode_MP"; CPWMMode "physmod:ee:library:comments:control:eePwmGeneratorTwoLevel:ContinuousPWM_MP"; DPWMMode "physmod:ee:library:comments:control:eePwmGeneratorTwoLevel:DiscontinuousPWM_MP"; SamplingMode "physmod:ee:library:comments:control:eePwmGeneratorTwoLevel:SamplingMode_MP"; fsw "physmod:ee:library:comments:control:eePwmGeneratorTwoLevel:SwitchingFrequencyHz_MP"; Ts "physmod:ee:library:comments:control:eePwmGeneratorTwoLevel:SampleTimes_MP"
      mask help: physmod:ee:library:comments:control:eePwmGeneratorTwoLevel:PWMGeneratorthreephaseTwolevel_MD
      mask init:
      | Tsw = 1/fsw;
      | 
      | if fsw <= 0
      |     error(message('physmod:simscape:compiler:patterns:checks:GreaterThanZero',getString(message('physmod:ee:library:comments:control:eePwmGeneratorTwoLevel:SwitchingFrequencyHz_MP'))));
      | end
      | 
      | if Ts <= 0
      |     error(message('physmod:simscape:compiler:patterns:checks:GreaterThanZero',getString(message('physmod:ee:library:comments:control:eePwmGeneratorTwoLevel:SampleTimes_MP'))));
      | end
      | 
      | if Ts > 1/(10*fsw)
      |     error(message('physmod:simscape:compiler:patterns:checks:LessThanOrEqual',getString(message('physmod:ee:library:comments:control:eePwmGeneratorTwoLevel:SampleTimes_MP')),getString(message('physmod:ee:library:comments:control:eePwmGeneratorTwoLevel:inverseOf10TimesSwitchingFrequency_MP'))));
      | end
      | 
      | switch SamplingMode
      |     case 'Natural'
      |         RateTransitionOnInput = -1;
      |         GateGeneratorX0 = 0;
      |     case 'Asymmetric'
      |         RateTransitionOnInput = 0.5*Tsw;
      |         GateGeneratorX0 = 0.5/fsw;
      |     case 'Symmetric'
      |         RateTransitionOnInput = Tsw;
      |         GateGeneratorX0 = 0;
      | end
      | 
      | 
      | switch PWMMode
      |     case 'Continuous PWM (CPWM)'
      |         switch CPWMMode
      |             case 'SPWM: sinusoidal PWM'
      |                 PWM = 1;
      |             case 'SVM: space vector modulation'
      |                 PWM = 2;
      |         end
      |     case 'Discontinuous PWM (DPWM)'
      |         switch DPWMMode
      |             case '60 DPWM: 60 degree discontinuous PWM'
      |                 PWM = 3;
      |             case '60 DPWM (+30 degree shift): +30 degree shift from 60 DPWM'
      |                 PWM = 4;
      |             case '60 DPWM (-30 degree shift): -30 degree shift from 60 DPWM'
      |                 PWM = 5;
      |             case '30 DPWM: 30 degree discontinuous PWM'
      |                 PWM = 6;
      |             case '120 DPWM: positive dc component'
      |                 PWM = 7;
      |             case '120 DPWM: negative dc component'
      |                 PWM = 8;
      |         end
      | end
      settings: CopyFcn=ee_sli_rtmsupport( 'copyfcn', gcbh );  DeleteFcn=ee_sli_rtmsupport( 'deletefcn', gcbh );  ModelCloseFcn=ee_sli_rtmsupport( 'modelclosefcn', gcbh );  PreSaveFcn=%pe_sli_rtmsupport( 'presavefcn', gcbh );  PostSaveFcn=ee_sli_rtmsupport( 'postsavefcn', gcbh );  PreCopyFcn=ee_sli_rtmsupport( 'precopyfcn', gcbh );  OpenFcn=ee_sli_rtmsupport( 'openfcn', gcbh );  CloseFcn=ee_sli_rtmsupport( 'closefcn', gcbh );  PreDeleteFcn=ee_sli_rtmsupport( 'predeletefcn', gcbh );
      mask Help: web(nesl_help(gcbh))
      mask TypeOptions PWMMode: physmod:ee:library:comments:control:eePwmGeneratorTwoLevel:ContinuousPWMCPWM_PV | physmod:ee:library:comments:control:eePwmGeneratorTwoLevel:DiscontinuousPWMDPWM_PV
      mask Callback PWMMode:
      | switch get_param(gcb,'PWMMode')
      |     case 'Continuous PWM (CPWM)'
      |         set_param(gcb,'MaskVisibilities',{'on';'on';'off';'on';'on';'on'})
      |     case 'Discontinuous PWM (DPWM)'
      |         set_param(gcb,'MaskVisibilities',{'on';'off';'on';'on';'on';'on'})
      | end
      mask TypeOptions CPWMMode: physmod:ee:library:comments:control:eePwmGeneratorTwoLevel:SPWMSinusoidalPWM_PV | physmod:ee:library:comments:control:eePwmGeneratorTwoLevel:SVMSpaceVectorModulation_PV
      mask TypeOptions DPWMMode: physmod:ee:library:comments:control:eePwmGeneratorTwoLevel:x60DPWM60DegreeDiscontinuousPWM_PV | physmod:ee:library:comments:control:eePwmGeneratorTwoLevel:x60DPWM30DegreeShift30DegreeShiftFrom60DPWM_PV | physmod:ee:library:comments:control:eePwmGeneratorTwoLevel:x60DPWM0x2D30DegreeShift0x2D30DegreeShiftFrom60DPWM_PV | physmod:ee:library:comments:control:eePwmGeneratorTwoLevel:x30DPWM30DegreeDiscontinuousPWM_PV | physmod:ee:library:comments:control:eePwmGeneratorTwoLevel:x120DPWMPositiveDcComponent_PV | physmod:ee:library:comments:control:eePwmGeneratorTwoLevel:x120DPWMNegativeDcComponent_PV
      mask TypeOptions SamplingMode: physmod:ee:library:comments:control:eePwmGeneratorTwoLevel:Natural_PV | physmod:ee:library:comments:control:eePwmGeneratorTwoLevel:Asymmetric_PV | physmod:ee:library:comments:control:eePwmGeneratorTwoLevel:Symmetric_PV
      mask DialogControl ParameterGroupVar Prompt: physmod:ee:library:comments:control:eePwmGeneratorTwoLevel:tab_Parameters
      mask DialogControl PWMMode Prompt: PWM mode
      mask DialogControl CPWMMode Prompt: Continuous PWM
      mask DialogControl DPWMMode Prompt: Discontinuous PWM
      mask DialogControl SamplingMode Prompt: Sampling mode
      mask DialogControl fsw Prompt: Switching frequency (Hz)
      mask DialogControl Ts Prompt: Sample time (s)
  Terminator : Terminator
  Terminator1 : Terminator
  ab2abc : Subsystem
  Vabc in PU : Outport  VectorParamsAs1DForOutWhenUnconnected=off
  wires:
  Inverse Park Transform/1 -> "PWM Generator (Three-phase, Two-level)"/1(Vabc)
  Mux/1 -> Inverse Park Transform/1
  "PWM Generator (Three-phase, Two-level)"/2(ModWave) -> Vabc in PU/1  "ModWave"
  "PWM Generator (Three-phase, Two-level)"/1(g) -> Terminator/1
  Constant1/1 -> "PWM Generator (Three-phase, Two-level)"/2(vdc)
  Constant/1 -> Mux/3
  Current_Controllers/2(Vq_ref) -> Mux/2
  Pos_PU/1 -> Clarke to Park Angle Transform/2, Inverse Park Transform/2
  Current_Controllers/1(Vd_ref) -> Mux/1
  Demux1/3 -> Terminator1/1
  Demux1/2 -> Current_Controllers/2(Iq)
  Demux1/1 -> Current_Controllers/1(Id)
  Clarke to Park Angle Transform/1 -> Demux1/1
  ab2abc/1(abc) -> Clarke Transform/1
  Iab_meas_PU/1 -> ab2abc/1(ab)
  Clarke Transform/1 -> Clarke to Park Angle Transform/1
  Idq_ref_PU/1 -> Current_Controllers/3(Idq_ref_PU)

== system Two_Zone_MVDC_PSolver/PGM1/Gas turbine/GAST/GAST/Subsystem ==
  u : Inport
  Discrete-Time Integrator : DiscreteIntegrator  SampleTime=TsCont  LimitOutput=on  UpperSaturationLimit=VMAX  LowerSaturationLimit=VMIN  ICPrevOutput=DiscIntNeverNeededParam  ICPrevScaledInput=DiscIntNeverNeededParam
  Gain2 : Gain  Gain=1/T
  Sum1 : Sum  Inputs=|+-
  y : Outport
  wires:
  Discrete-Time Integrator/1 -> y/1, Sum1/2
  Gain2/1 -> Discrete-Time Integrator/1
  Sum1/1 -> Gain2/1
  u/1 -> Sum1/1

== system Two_Zone_MVDC_PSolver/PGM1/Gas turbine/GAST/GAST/Subsystem1 ==
  u : Inport
  Discrete-Time Integrator : DiscreteIntegrator  SampleTime=TsCont  LimitOutput=on  UpperSaturationLimit=VMAX  LowerSaturationLimit=VMIN  ICPrevOutput=DiscIntNeverNeededParam  ICPrevScaledInput=DiscIntNeverNeededParam
  Gain2 : Gain  Gain=1/T
  Sum1 : Sum  Inputs=|+-
  y : Outport
  wires:
  u/1 -> Sum1/1
  Sum1/1 -> Gain2/1
  Gain2/1 -> Discrete-Time Integrator/1
  Discrete-Time Integrator/1 -> Sum1/2, y/1

== system Two_Zone_MVDC_PSolver/PGM1/Gas turbine/GAST/GAST/Subsystem2 ==
  u : Inport
  Discrete-Time Integrator : DiscreteIntegrator  SampleTime=TsCont  LimitOutput=on  UpperSaturationLimit=VMAX  LowerSaturationLimit=VMIN  ICPrevOutput=DiscIntNeverNeededParam  ICPrevScaledInput=DiscIntNeverNeededParam
  Gain2 : Gain  Gain=1/T
  Sum1 : Sum  Inputs=|+-
  y : Outport
  wires:
  Discrete-Time Integrator/1 -> y/1, Sum1/2
  Gain2/1 -> Discrete-Time Integrator/1
  Sum1/1 -> Gain2/1
  u/1 -> Sum1/1

== system Two_Zone_MVDC_PSolver/PGM2/Gas turbine/GAST/GAST/Subsystem ==
  u : Inport
  Discrete-Time Integrator : DiscreteIntegrator  SampleTime=TsCont  LimitOutput=on  UpperSaturationLimit=VMAX  LowerSaturationLimit=VMIN  ICPrevOutput=DiscIntNeverNeededParam  ICPrevScaledInput=DiscIntNeverNeededParam
  Gain2 : Gain  Gain=1/T
  Sum1 : Sum  Inputs=|+-
  y : Outport
  wires:
  Discrete-Time Integrator/1 -> y/1, Sum1/2
  Gain2/1 -> Discrete-Time Integrator/1
  Sum1/1 -> Gain2/1
  u/1 -> Sum1/1

== system Two_Zone_MVDC_PSolver/PGM2/Gas turbine/GAST/GAST/Subsystem1 ==
  u : Inport
  Discrete-Time Integrator : DiscreteIntegrator  SampleTime=TsCont  LimitOutput=on  UpperSaturationLimit=VMAX  LowerSaturationLimit=VMIN  ICPrevOutput=DiscIntNeverNeededParam  ICPrevScaledInput=DiscIntNeverNeededParam
  Gain2 : Gain  Gain=1/T
  Sum1 : Sum  Inputs=|+-
  y : Outport
  wires:
  u/1 -> Sum1/1
  Sum1/1 -> Gain2/1
  Gain2/1 -> Discrete-Time Integrator/1
  Discrete-Time Integrator/1 -> Sum1/2, y/1

== system Two_Zone_MVDC_PSolver/PGM2/Gas turbine/GAST/GAST/Subsystem2 ==
  u : Inport
  Discrete-Time Integrator : DiscreteIntegrator  SampleTime=TsCont  LimitOutput=on  UpperSaturationLimit=VMAX  LowerSaturationLimit=VMIN  ICPrevOutput=DiscIntNeverNeededParam  ICPrevScaledInput=DiscIntNeverNeededParam
  Gain2 : Gain  Gain=1/T
  Sum1 : Sum  Inputs=|+-
  y : Outport
  wires:
  Discrete-Time Integrator/1 -> y/1, Sum1/2
  Gain2/1 -> Discrete-Time Integrator/1
  Sum1/1 -> Gain2/1
  u/1 -> Sum1/1

== system Two_Zone_MVDC_PSolver/PMM/Control/Torque Control/Control_System/Current_Controllers ==
  Id : Inport
  Iq : Inport  Port=2
  Idq_ref_PU : Inport  Port=3
  Demux : Demux  Outputs=2
  PI_Controller_Id : Subsystem
  PI_Controller_Iq : Subsystem
  Vd_ref : Outport  VectorParamsAs1DForOutWhenUnconnected=off
  Vq_ref : Outport  Port=2  VectorParamsAs1DForOutWhenUnconnected=off
  wires:
  Demux/2 -> PI_Controller_Iq/1(I_ref)
  Demux/1 -> PI_Controller_Id/1(I_ref)
  PI_Controller_Iq/1(V_ref) -> Vq_ref/1
  PI_Controller_Id/1(V_ref) -> Vd_ref/1
  Idq_ref_PU/1 -> Demux/1
  Id/1 -> PI_Controller_Id/2(I_fb)
  Iq/1 -> PI_Controller_Iq/2(I_fb)

== system Two_Zone_MVDC_PSolver/PMM/Control/Torque Control/Control_System/PWM Generator (Three-phase, Two-level) ==
  Vabc : Inport
  vdc : Inport  Port=2
  Data Type Conversion : DataTypeConversion  SaturateOnIntegerOverflow=off  RndMeth=Floor
  Data Type Conversion1 : DataTypeConversion  SaturateOnIntegerOverflow=off  RndMeth=Floor
  Gate Signal Generator : Subsystem
  RTabc : RateTransition  Deterministic=off  OutPortSampleTime=RateTransitionOnInput
  RTdc : RateTransition  Deterministic=off  OutPortSampleTime=RateTransitionOnInput
  Switching Time Calculation : MATLAB Function  TreatAsAtomicUnit=on
  avoid division by 0 : Saturate  UpperLimit=inf  LowerLimit=eps
  g : Outport  VectorParamsAs1DForOutWhenUnconnected=off
  ModWave : Outport  Port=2  VectorParamsAs1DForOutWhenUnconnected=off
  wires:
  Data Type Conversion1/1 -> ModWave/1
  avoid division by 0/1 -> Switching Time Calculation/2(vdc)
  RTdc/1 -> avoid division by 0/1
  RTabc/1 -> Switching Time Calculation/1(Vabc)
  Switching Time Calculation/3(ModWave) -> Data Type Conversion1/1
  Data Type Conversion/1 -> g/1
  Gate Signal Generator/1(s) -> Data Type Conversion/1
  Switching Time Calculation/2(TgabcOFF) -> Gate Signal Generator/2(TgabcOFF)
  Switching Time Calculation/1(TgabcON) -> Gate Signal Generator/1(TgabcON)
  Vabc/1 -> RTabc/1
  vdc/1 -> RTdc/1

== system Two_Zone_MVDC_PSolver/PMM/Control/Torque Control/Control_System/ab2abc ==
  ab : Inport
  Demux1 : Demux  Outputs=2
  Mux : Mux  Inputs=3
  Sum : Sum  Inputs=--
  abc : Outport
  wires:
  ab/1 -> Demux1/1
  Demux1/2 -> Mux/2, Sum/1
  Sum/1 -> Mux/3
  Mux/1 -> abc/1
  Demux1/1 -> Mux/1, Sum/2
